simulink model "Transformada_de_Park_inversa"  (R2021a)
settings: Solver=VariableStepAuto  StartTime=0.0  StopTime=10.0  RelTol=1e-3
settings Model: Creator=fhlla  LastModifiedBy=fhlla

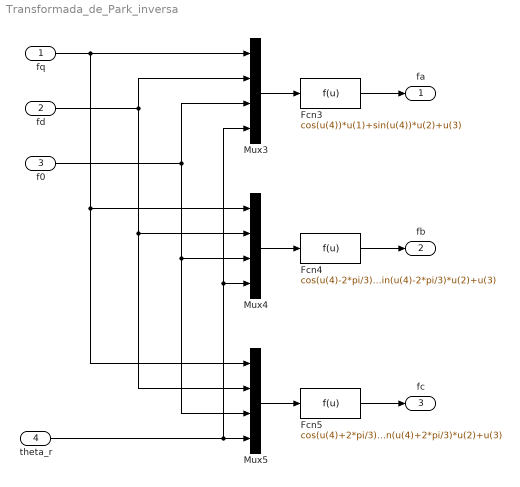
== system Transformada_de_Park_inversa ==
  fq : Inport
  fd : Inport  Port=2
  f0 : Inport  Port=3
  theta_r : Inport  Port=4
  Fcn3 : Fcn  Expr=cos(u(4))*u(1)+sin(u(4))*u(2)+u(3)
  Fcn4 : Fcn  Expr=cos(u(4)-2*pi/3)*u(1)+sin(u(4)-2*pi/3)*u(2)+u(3)
  Fcn5 : Fcn  Expr=cos(u(4)+2*pi/3)*u(1)+sin(u(4)+2*pi/3)*u(2)+u(3)
  Mux3 : Mux
  Mux4 : Mux
  Mux5 : Mux
  fa : Outport
  fb : Outport  Port=2
  fc : Outport  Port=3
  wires:
  Mux5/1 -> Fcn5/1
  Fcn5/1 -> fc/1
  fd/1 -> Mux5/2, Mux4/2, Mux3/2
  Mux3/1 -> Fcn3/1
  Mux4/1 -> Fcn4/1
  Fcn4/1 -> fb/1
  fq/1 -> Mux3/1, Mux5/1, Mux4/1
  Fcn3/1 -> fa/1
  theta_r/1 -> Mux3/4, Mux4/4, Mux5/4
  f0/1 -> Mux5/3, Mux4/3, Mux3/3
